simulink model "Mrac_IeI"  (R2021a)
settings: Solver=VariableStepAuto  StartTime=0.0  StopTime=50  RelTol=1e-3
settings Model: Creator=simon  LastModifiedBy=simon

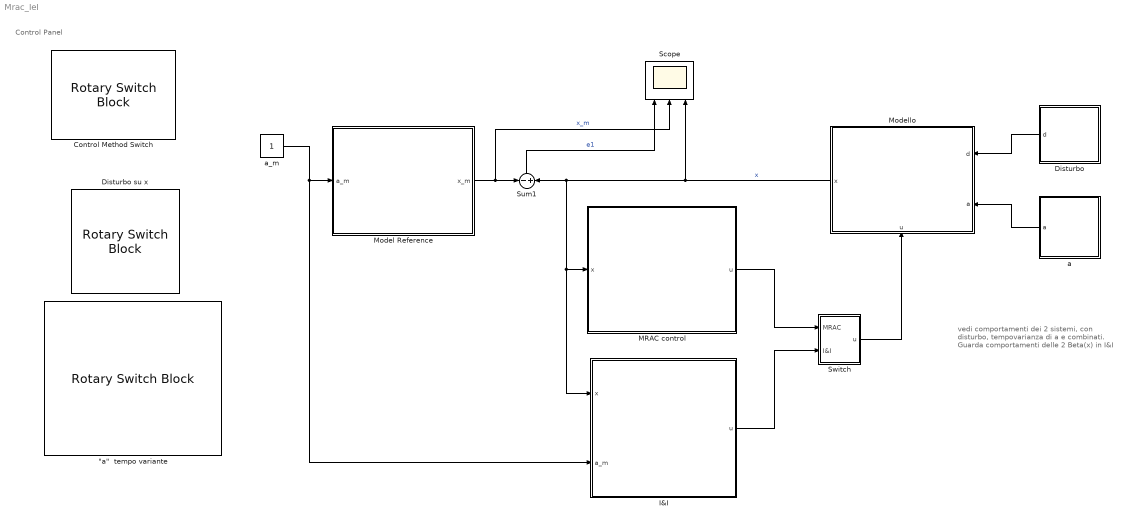
== system Mrac_IeI ==
  note: Control Panel
  note: vedi comportamenti dei 2 sistemi, con
      | disturbo, tempovarianza di a e combinati.
      | Guarda comportamenti delle 2 Beta(x)
      | in I&I
  "\"a\"  tempo variante" : RotarySwitchBlock  LabelPosition=Hide
      settings: Values={{'Cost', '1/10sin(10t)', '10sin(t/10)'}, [3 1 2]}
  Control Method Switch : RotarySwitchBlock  LabelPosition=Hide
      settings: Values={{'MRAC', 'I&I'}, [1 2]}
  Disturbo : Subsystem
  Disturbo su x : RotarySwitchBlock  LabelPosition=Hide
      settings: Values={{'Off', 'On'}, [2 1]}
  I&I : Subsystem
  MRAC control : Subsystem
  Model Reference : Subsystem
  "Modello " : Subsystem
      settings: PortSchema="{\"entries\":[{\"content\":{\"sides\":[{\"content\":{\"connectorIds\":[\"In1\",\"In2\"]},\"type\":\"ConnectorPlacement.EquallySpacedRectSide\",\"uuid\":\"60128dcc-c94e-4ce3-afb1-22f906940115\"},{\"content\":{\"connectorIds\":[\"Out1\"],\"side\":\"RIGHT\"},\"type\":\"ConnectorPlacement.EquallySpacedRectSide\",\"uuid\":\"9e4146dc-925c-4f3e-99b3-a5904ff107a3\"},{\"content\":{\"connectorIds\":[],\"side\":\"TOP\"},\"type\":\"ConnectorPlacement.EquallySpacedRectSide\",\"uuid\":\"39f32b01-25e6-41dd-9c0f-353a8d1eb187\"},{\"content\":{\"connectorIds\":[\"In3\"],\"side\":\"BOTTOM\"},\"type\":\"ConnectorPlacement.EquallySpacedRectSide\",\"uuid\":\"352c59dd-08a6-4aa7-aece-93859692fa6f\"}]},\"type\":\"ConnectorPlacement.EquallySpacedConnector\",\"uuid\":\"b6a33f77-7c3a-4f7b-932f-c7361b7e2bf3\"}],\"packageUris\":[\"http://schema.mathworks.com/mf0/Connector/R2020b\"],\"version\":\"1.0\"}"
  Scope : Scope  NumInputPorts=3
  Sum1 : Sum  Inputs=-+
  Switch : Subsystem
  a : Subsystem
  a_m : Constant
  wires:
  a_m/1 -> Model Reference/1(a_m), I&I/2(a_m)
  Model Reference/1(x_m) -> Scope/2, Sum1/1  "x_m"
  MRAC control/1(u) -> Switch/1(MRAC)
  I&I/1(u) -> Switch/2(I&I)
  "Modello "/1(x) -> Scope/3, MRAC control/1(x), I&I/1(x), Sum1/2  "x"
  Disturbo/1(d) -> "Modello "/1(d)
  Switch/1(u) -> "Modello "/3(u)
  a/1(a) -> "Modello "/2(a)
  Sum1/1 -> Scope/1  "e1"

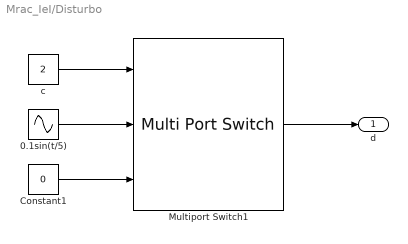
== system Mrac_IeI/Disturbo ==
  0.1sin(t/5) : Sin  Amplitude=0.1  Frequency=1/5  SampleTime=0
  Constant1 : Constant  Value=0
  Multiport Switch1 : MultiPortSwitch  Inputs=2
  c : Constant  Value=2
  d : Outport
  wires:
  c/1 -> Multiport Switch1/1
  0.1sin(t/5)/1 -> Multiport Switch1/2
  Multiport Switch1/1 -> d/1
  Constant1/1 -> Multiport Switch1/3

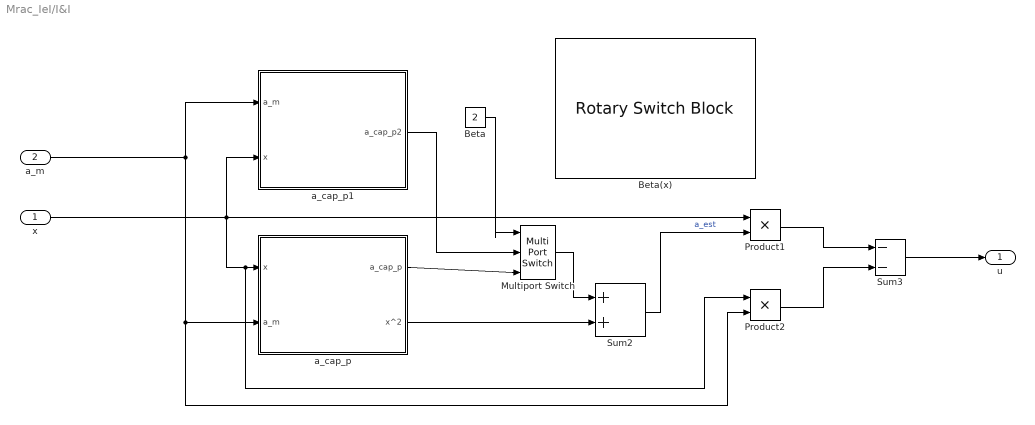
== system Mrac_IeI/I&I ==
  x : Inport
  a_m : Inport  Port=2
  Beta : Constant  Value=2
  Beta(x) : RotarySwitchBlock  LabelPosition=Hide
      settings: Values={{'(x^2)/2', '1/2log(1+x^2)'}, [2 1]}
  Multiport Switch : MultiPortSwitch  Inputs=2
  Product1 : Product
  Product2 : Product
  Sum2 : Sum
  Sum3 : Sum  Inputs=--
  a_cap_p : Subsystem
  a_cap_p1 : Subsystem
  u : Outport
  wires:
  Product2/1 -> Sum3/2
  a_cap_p/2(x^2) -> Sum2/2
  Sum2/1 -> Product1/2  "a_est"
  Product1/1 -> Sum3/1
  Sum3/1 -> u/1
  a_m/1 -> a_cap_p1/1(a_m), a_cap_p/2(a_m), Product2/2
  x/1 -> a_cap_p/1(x), Product2/1, Product1/1, a_cap_p1/2(x)
  a_cap_p/1(a_cap_p) -> Multiport Switch/3
  Multiport Switch/1 -> Sum2/1
  a_cap_p1/1(a_cap_p2) -> Multiport Switch/2
  Beta/1 -> Multiport Switch/1

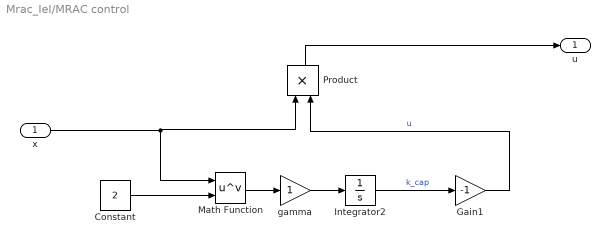
== system Mrac_IeI/MRAC control ==
  x : Inport
  Constant : Constant  Value=2
  Gain1 : Gain  Gain=-1
  Integrator2 : Integrator  InitialCondition=1
  Math Function : Math  Operator=pow  SaturateOnIntegerOverflow=on
  Product : Product
  gamma : Gain
  u : Outport
  wires:
  Math Function/1 -> gamma/1
  Constant/1 -> Math Function/2
  Integrator2/1 -> Gain1/1  "k_cap"
  gamma/1 -> Integrator2/1
  x/1 -> Product/1, Math Function/1
  Gain1/1 -> Product/2  "u"
  Product/1 -> u/1

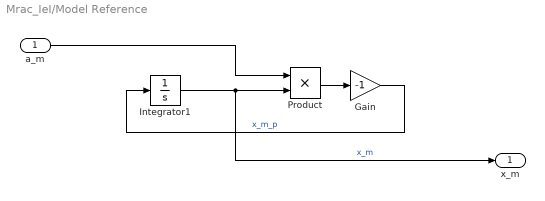
== system Mrac_IeI/Model Reference ==
  a_m : Inport
  Gain : Gain  Gain=-1
  Integrator1 : Integrator  InitialCondition=2
  Product : Product
  x_m : Outport
  wires:
  Integrator1/1 -> x_m/1, Product/2  "x_m"
  Gain/1 -> Integrator1/1  "x_m_p"
  Product/1 -> Gain/1
  a_m/1 -> Product/1

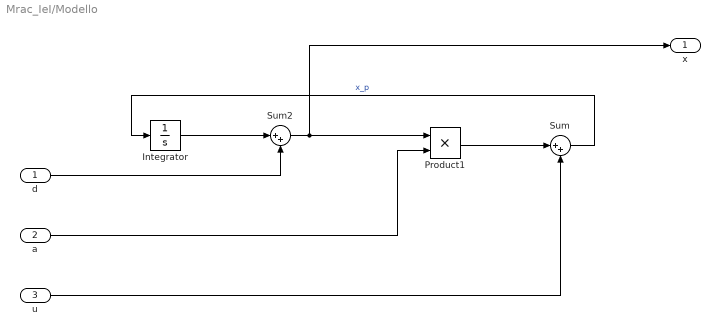
== system Mrac_IeI/Modello  ==
  d : Inport
  a : Inport  Port=2
  u : Inport  Port=3
  Integrator : Integrator  InitialCondition=2
  Product1 : Product
  Sum : Sum  Inputs=|++
  Sum2 : Sum  Inputs=|++
  x : Outport
  wires:
  d/1 -> Sum2/2
  Sum/1 -> Integrator/1  "x_p"
  u/1 -> Sum/2
  Sum2/1 -> Product1/1, x/1
  a/1 -> Product1/2
  Integrator/1 -> Sum2/1
  Product1/1 -> Sum/1

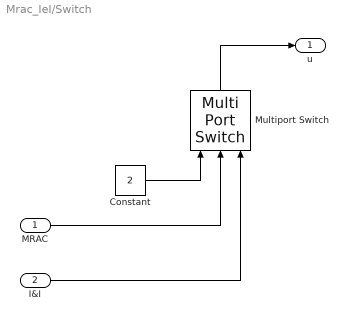
== system Mrac_IeI/Switch ==
  MRAC : Inport
  I&I : Inport  Port=2
  Constant : Constant  Value=2
  Multiport Switch : MultiPortSwitch  Inputs=2
  u : Outport
  wires:
  MRAC/1 -> Multiport Switch/2
  Constant/1 -> Multiport Switch/1
  Multiport Switch/1 -> u/1
  I&I/1 -> Multiport Switch/3

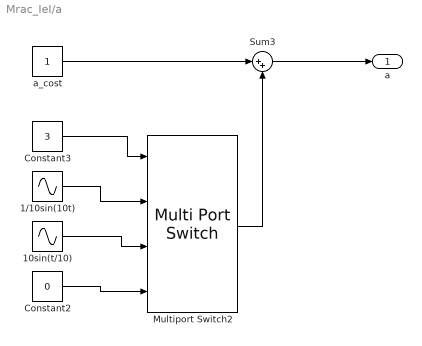
== system Mrac_IeI/a ==
  1/10sin(10t) : Sin  Amplitude=1/10  Frequency=10  SampleTime=0
  10sin(t/10) : Sin  Amplitude=10  Frequency=1/10  SampleTime=0
  Constant2 : Constant  Value=0
  Constant3 : Constant  Value=3
  Multiport Switch2 : MultiPortSwitch
  Sum3 : Sum  Inputs=|++
  a_cost : Constant
  a : Outport
  wires:
  Sum3/1 -> a/1
  a_cost/1 -> Sum3/1
  Multiport Switch2/1 -> Sum3/2
  Constant3/1 -> Multiport Switch2/1
  Constant2/1 -> Multiport Switch2/4
  1/10sin(10t)/1 -> Multiport Switch2/2
  10sin(t/10)/1 -> Multiport Switch2/3

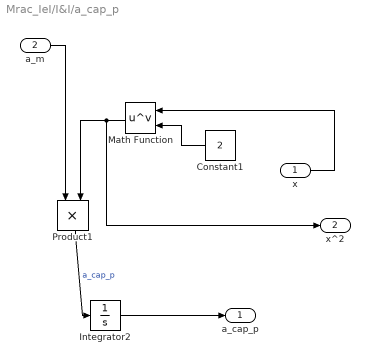
== system Mrac_IeI/I&I/a_cap_p ==
  x : Inport
  a_m : Inport  Port=2
  Constant1 : Constant  Value=2
  Integrator2 : Integrator
  Math Function : Math  Operator=pow  SaturateOnIntegerOverflow=on
  Product1 : Product
  a_cap_p : Outport
  x^2 : Outport  Port=2
  wires:
  Math Function/1 -> x^2/1, Product1/2
  Constant1/1 -> Math Function/2
  a_m/1 -> Product1/1
  Integrator2/1 -> a_cap_p/1
  Product1/1 -> Integrator2/1  "a_cap_p"
  x/1 -> Math Function/1

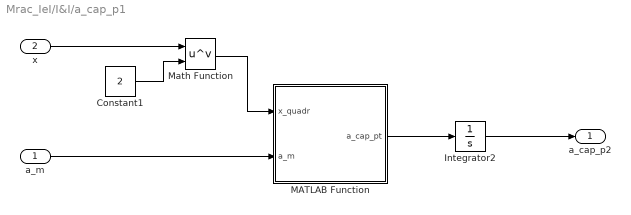
== system Mrac_IeI/I&I/a_cap_p1 ==
  a_m : Inport
  x : Inport  Port=2
  Constant1 : Constant  Value=2
  Integrator2 : Integrator
  MATLAB Function : MATLAB Function  TreatAsAtomicUnit=on
  Math Function : Math  Operator=pow  SaturateOnIntegerOverflow=on
  a_cap_p2 : Outport
  wires:
  Math Function/1 -> MATLAB Function/1(x_quadr)
  Constant1/1 -> Math Function/2
  a_m/1 -> MATLAB Function/2(a_m)
  Integrator2/1 -> a_cap_p2/1
  x/1 -> Math Function/1
  MATLAB Function/1(a_cap_pt) -> Integrator2/1

== matlab function Mrac_IeI/I&I/a_cap_p1/MATLAB Function ==
  data: x_quadr input; a_m input; a_cap_pt output
function a_cap_pt = fcn(x_quadr, a_m)

a_cap_pt = (a_m*x_quadr)/(1+x_quadr);
